simulink model "CF018A_GmRoadWhlInQlfr"  (R2013b)
settings: Solver=FixedStepDiscrete  SolverMode=SingleTasking  StartTime=0.0  StopTime=1  FixedStep=0.002  RelTol=1e-3
values from neighbouring files (symbols this model uses):
  DELTAPLSROLLOVR_CNT_S16 = DataDict.Constant    [CF018A_GmRoadWhlInQlfr_DataDict.m]
  DELTATISTAMPCNTROLLOVR_CNT_S32 = DataDict.Constant    [CF018A_GmRoadWhlInQlfr_DataDict.m]
  GmRoadWhlInQlfrMaxAllwblFrq = DataDict.Calibration    [CF018A_GmRoadWhlInQlfr_DataDict.m]
  GmRoadWhlInQlfrMaxFrqChg = DataDict.Calibration    [CF018A_GmRoadWhlInQlfr_DataDict.m]
  LEFRQCHGOUTOFRNG_CNT_U08 = DataDict.Constant    [CF018A_GmRoadWhlInQlfr_DataDict.m]
  LEFRQOUTOFRNG_CNT_U08 = DataDict.Constant    [CF018A_GmRoadWhlInQlfr_DataDict.m]
  NODEBSTEP_CNT_U16 = DataDict.Constant    [CF018A_GmRoadWhlInQlfr_DataDict.m]
  PARKDURN_CNT_F32 = DataDict.Constant    [CF018A_GmRoadWhlInQlfr_DataDict.m]
  PREVRAWWHLFRQMIN_HZ_F32 = DataDict.Constant    [CF018A_GmRoadWhlInQlfr_DataDict.m]
  RIFRQCHGOUTOFRNG_CNT_U08 = DataDict.Constant    [CF018A_GmRoadWhlInQlfr_DataDict.m]
  RIFRQOUTOFRNG_CNT_U08 = DataDict.Constant    [CF018A_GmRoadWhlInQlfr_DataDict.m]
  RoadWhlFrqInCalcOutOfRng = DataDict.NTC    [CF018A_GmRoadWhlInQlfr_DataDict.m]
  SECTO100MICROSECCNVN_CNT_F32 = DataDict.Constant    [CF018A_GmRoadWhlInQlfr_DataDict.m]
  WHLFRQMIN_HZ_F32 = DataDict.Constant    [CF018A_GmRoadWhlInQlfr_DataDict.m]
undefined symbols (not defined in the file or in its folder): NtcSts1
libraries: simulink x5, NxtrAbslt x2, NxtrLim x2
(part 1 of 5)
settings Model: PauseTimes=2  CovMetricSettings=dcmrw  CovFilter=CF09_GMOverlayStateHandler_v002_covfilter  CovHTMLOptions=-sRT=1 -aTS=1 -bRG=1 -bTC=1 -hTR=0 -nFC=0 -scm=1 -bcm=1 -xEv=0  covSaveCumulativeToWorkspaceVar=off  CovSaveSingleToWorkspaceVar=off  CovCumulativeReport=on  Creator=SZ7VY6  LastModifiedBy=BZHF94
settings SolverCC: AutoInsertRateTranBlk=on  InsertRTBMode=Always
settings DataIOCC: LimitDataPoints=off  SaveFormat=Structure  ReturnWorkspaceOutputs=on
settings OptimizationCC: BlockReduction=off  InlineParams=on  ZeroExternalMemoryAtStartup=off  ZeroInternalMemoryAtStartup=off  OptimizeModelRefInitCode=on  LifeSpan=1
settings DebuggingCC: SignalInfNanChecking=error  SignalRangeChecking=warning  UnderspecifiedInitializationDetection=Simplified  SolverPrmCheckMsg=error  InheritedTsInSrcMsg=error  DiscreteInheritContinuousMsg=error  SingleTaskRateTransMsg=error  TasksWithSamePriorityMsg=error  SigSpecEnsureSampleTimeMsg=error  CheckMatrixSingularityMsg=error  ParameterUnderflowMsg=error  ParameterPrecisionLossMsg=error  ParameterTunabilityLossMsg=error  FixptConstUnderflowMsg=warning  FixptConstOverflowMsg=warning  VectorMatrixConversionMsg=error  SignalLabelMismatchMsg=error  UnconnectedInputMsg=error  UnconnectedOutputMsg=error  UnconnectedLineMsg=error  SFcnCompatibilityMsg=error  UniqueDataStoreMsg=warning  BusObjectLabelMismatch=error  RootOutportRequireBusObject=error  AssertControl=DisableAll  ModelReferenceIOMsg=error  ModelReferenceVersionMismatchMessage=warning  ModelReferenceIOMismatchMessage=error  ModelReferenceCSMismatchMessage=warning  ModelReferenceDataLoggingMessage=error  StateNameClashWarn=warning  StrictBusMsg=ErrorOnBusTreatedAsVector  NonBusSignalsTreatedAsBus=error  SFUnexpectedBacktrackingDiag=error  SFInvalidInputDataAccessInChartInitDiag=error  SFNoUnconditionalDefaultTransitionDiag=error  SFTransitionOutsideNaturalParentDiag=error  SFUnconditionalTransitionShadowingDiag=error  SFUndirectedBroadcastEventsDiag=error
settings ModelReferenceCC: ModelReferenceNumInstancesAllowed=Single
settings RTWCC: SystemTargetFile=autosar.tlc  GenCodeOnly=on  TemplateMakefile=ert_default_tmf  Description=AUTOSAR  GenerateReport=on  ProcessScript=autosar_make_rtw_hook  LaunchReport=on
settings CodeAppCC: GenerateComments=off  IgnoreCustomStorageClasses=off  CustomSymbolStrType=$N$R$M  CustomSymbolStrBlkIO=$N$M  SimulinkBlockComments=off
settings STFCustomTargetCC: ParMdlRefBuildCompliant=on  CompOptLevelCompliant=on  IncludeMdlTerminateFcn=off  CombineOutputUpdateFcns=on  SuppressErrorStatus=on  ERTFirstTimeCompliant=on  ERTCustomFileBanners=on  SupportNonFinite=off  SupportComplex=off  SupportContinuousTime=off  SupportNonInlinedSFcns=off  MATLABClassNameForMDSCustomization=Simulink.SoftwareTarget.ERTCustomization  AutosarCompliant=on  GRTInterface=off  SystemTargetFile=autosar.tlc
settings ERTTargetCC: CodeReplacementLibrary=ANSI_C  ConcurrentExecutionCompliant=off  IncludeMdlTerminateFcn=off  SuppressErrorStatus=on  SupportNonFinite=off  SupportComplex=off  ModelStepFunctionPrototypeControlCompliant=off  CPPClassGenCompliant=off  AutosarCompliant=on  InlinedParameterPlacement=NonHierarchical  ERTCustomFileTemplate=example_file_process.tlc  EnableUserReplacementTypes=on

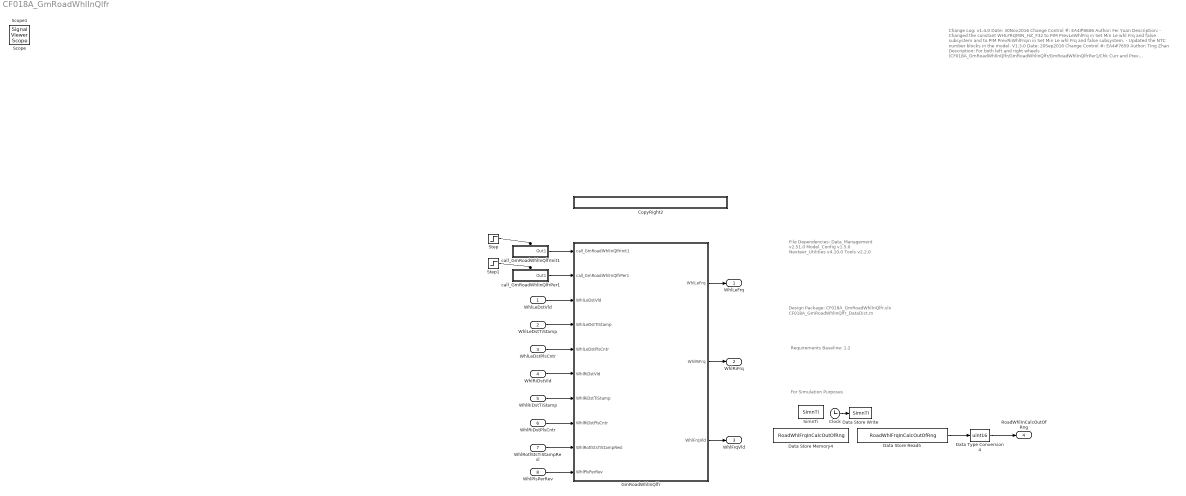
== system CF018A_GmRoadWhlInQlfr ==
  note: File Dependencies:
      |
      | Data_Management v2.51.0
      | Model_Config v1.5.0
      | Nexteer_Utilities v4.10.0
      | Tools v2.2.0
  note: Requirements Baseline: 1.2
  note: Change Log:
      |
      | v1.4.0
      | Date: 30Nov2016
      | Change Control #: EA4#8606
      | Author: Fei Yuan
      | Description:
      | - Changed the constant WHLFRQMIN_HZ_F32 to PIM PrevLeWhlFrq in
      |   Set Min Le whl Frq and false subsystem and to PIM PrevRiWhlFrqin  in
      |   Set Min Le whl Frq and false subsystem.
      | - Updated the NTC number blocks in the model.
      |
      |
      | V1.3.0
      | Date: 20Sep2016
      | Change Control #: EA4#7659
      | Author: Ting Zhan
      | Description:
      | For both left and right wheels (CF018A_GmRoadWhlInQlfr/GmRoadWhlInQlfr/GmRoadWhlInQlfrPer1/Chk Curr and Prev LeWhlDstTiStamp/Calc LeWhlFrq and LeWhlFrqVld /Calc
      | LeWhlFrq and LeWhlFrqVld and the corresponding right wheel block.)
      | 1.Adjust the math in the local processing functions to
      | cast to a sint32/sin16 before subtracting the timestampts/counters to produce the deltatistamp/deltacntr
      | 2.Move conversions before caluculating RawLeWhlFrq_WhlRevPerSec_T_F32 to avoid rollover
      |
      | V1.2.0
      | Date: 20Sep2016
      | Change Control #: EA4#4919
      | Author: Ting Zhan
      | Description:
      | -Added display variables dGmRoadWhlInQlrRawLeWhlFrq, dGmRoadWhlInQlrRawRiWhlFrq,
      |  dGmRoadWhlInQlrRawLeDeltaPls, dGmRoadWhlInQlrRawRiDeltaPls,
      |  dGmRoadWhlInQlrLeDeltaTiStamp, and dGmRoadWhlInQlrRiDeltaTiStamp
      | -Moved uint16 conversion after summation
      | -Changed time steps in .m file
      |
      | V 1.1.0
      | Date: 03Mar2016
      | Change Control #: EA4#7312
      | Author: Ting Zhan
      | Description:
      | - Added constant PREVRAWWHLFRQMIN_HZ_F32 in .m file
      |
      | V 1.0.0
      | Date: 22Feb2016
      | Change Control #: EA4#3951
      | Author: Ting Zhan
      | Description:
      | - Initial Release Based on EA4
      | CR Number: 3951
  note: For Simulation Purposes
  note: Design Package:
      | CF018A_GmRoadWhlInQlfr.slx
      | CF018A_GmRoadWhlInQlfr_DataDict.m
  WhlLeDstVld : Inport  RequirementInfo={} %GIDa_1b9c6812_2c02_4b85_9a2c_669458cc48bb  OutDataTypeStr=boolean
  WhlLeDstTiStamp : Inport  RequirementInfo={} %GIDa_61858a6e_79fe_432d_a90a_cf452097a93f  Port=2  OutDataTypeStr=uint16
  WhlLeDstPlsCntr : Inport  RequirementInfo={} %GIDa_f6a8d43a_8d7a_4621_b19c_bbf61fc3f1fb  Port=3  OutDataTypeStr=uint16
  WhlRiDstVld : Inport  RequirementInfo={} %GIDa_22f98033_b4f5_42bb_8f03_a53bfeb234c8  Port=4  OutDataTypeStr=boolean
  WhlRiDstTiStamp : Inport  RequirementInfo={} %GIDa_7d9397bd_97c2_42df_a94b_20b8f742e3e0  Port=5  OutDataTypeStr=uint16
  WhlRiDstPlsCntr : Inport  RequirementInfo={} %GIDa_8fb663a6_7a2b_45c8_868b_fc9c2da216fb  Port=6  OutDataTypeStr=uint16
  WhlRotlStsTiStampResl : Inport  RequirementInfo={} %GIDa_c41d293e_2c9d_4d75_aad1_09b36476f615  Port=7  OutDataTypeStr=single
  WhlPlsPerRev : Inport  RequirementInfo={} %GIDa_1e446983_1b59_4eb5_9ec1_824701f5829e  Port=8  OutDataTypeStr=uint8
  Clock : Clock
  CopyRight2 : Subsystem  Description=|  mask(Copyright Information){none=on}
      | Copyright info block.                                               
      |                                                                     
      | Place copyright information at the top of every subsystem in design.
      mask prompts: none "No parameters"
      mask help: Place copyright information at the top of every subsystem in design.
      mask Display:
      | NxtrConf = 'Nexteer Confidential';
      | 
      | sys = bdroot; %handle for the current model ("system")
      | first = get_param(sys,'Created');
      | if(isempty(first))
      |     first = datestr(now,'yyyy');
      | else
      |     first = first(end-3:end);  %year is last four digits
      | end
      | 
      | last = get_param(sys,'LastModifiedDate');
      | if isempty(last)
      |     last = datestr(now,'yyyy');
      | else
      |     last = last(end-3:end);
      | end
      | 
      | if strcmp(first,last)
      |     fprintf('%s -- Copyright %s Nexteer',NxtrConf,first)
      | else
      |     fprintf('%s -- %s%s- %s Nexteer',NxtrConf,char(169),first,last)
      | end
  Data Store Memory4 : DataStoreMemory  DataStoreName=RoadWhlFrqInCalcOutOfRng  InitialValue=NtcSts1.NTCSTS_PASSD  OutDataTypeStr=Enum: NtcSts1
  Data Store Read5 : DataStoreRead  DataStoreName=RoadWhlFrqInCalcOutOfRng  SampleTime=.004
  Data Store Write : DataStoreWrite  DataStoreName=SimnTi
  Data Type Conversion4 : DataTypeConversion  OutDataTypeStr=uint16
  GmRoadWhlInQlfr : Subsystem
  SimnTi : DataStoreMemory  DataStoreName=SimnTi
  Step : Step  Time=.001  Before=1  After=0  SampleTime=0
  Step1 : Step  Time=0.002  SampleTime=0
  call_GmRoadWhlInQlfrInit1 : Subsystem  TreatAsAtomicUnit=on
  call_GmRoadWhlInQlfrPer1 : Subsystem  TreatAsAtomicUnit=on
  WhlLeFrq : Outport  RequirementInfo={} %GIDa_1da87020_2114_47f8_bd6a_dcf122c70ef9
  WhlRiFrq : Outport  RequirementInfo={} %GIDa_aa71e542_5f04_4ff7_aa01_7ea85d72a732  Port=2
  WhlFrqVld : Outport  RequirementInfo={} %GIDa_6ce0db0a_f918_4040_a381_a66b37fb6372  Port=3
  RoadWhlInCalcOutOfRng : Outport  RequirementInfo={} %GIDa_f8f24313_b0b7_4842_bede_f0c570d36cae  Port=4
  Scope : SignalViewerScope  IOType=viewer  RefreshTime=0.035000
  Scope1 : SignalViewerScope  IOType=viewer  RefreshTime=0.035000
  wires:
  Step/1 -> call_GmRoadWhlInQlfrInit1/Enable
  call_GmRoadWhlInQlfrInit1/1(Out1) -> GmRoadWhlInQlfr/1(call_GmRoadWhlInQlfrInit1)
  Clock/1 -> Data Store Write/1
  GmRoadWhlInQlfr/2(WhlRiFrq) -> WhlRiFrq/1
  GmRoadWhlInQlfr/1(WhlLeFrq) -> WhlLeFrq/1
  Step1/1 -> call_GmRoadWhlInQlfrPer1/Enable
  call_GmRoadWhlInQlfrPer1/1(Out1) -> GmRoadWhlInQlfr/2(call_GmRoadWhlInQlfrPer1)
  GmRoadWhlInQlfr/3(WhlFrqVld) -> WhlFrqVld/1
  Data Store Read5/1 -> Data Type Conversion4/1
  Data Type Conversion4/1 -> RoadWhlInCalcOutOfRng/1
  WhlLeDstVld/1 -> GmRoadWhlInQlfr/3(WhlLeDstVld)
  WhlLeDstPlsCntr/1 -> GmRoadWhlInQlfr/5(WhlLeDstPlsCntr)
  WhlLeDstTiStamp/1 -> GmRoadWhlInQlfr/4(WhlLeDstTiStamp)
  WhlPlsPerRev/1 -> GmRoadWhlInQlfr/10(WhlPlsPerRev)
  WhlRiDstVld/1 -> GmRoadWhlInQlfr/6(WhlRiDstVld)
  WhlRiDstTiStamp/1 -> GmRoadWhlInQlfr/7(WhlRiDstTiStamp)
  WhlRiDstPlsCntr/1 -> GmRoadWhlInQlfr/8(WhlRiDstPlsCntr)
  WhlRotlStsTiStampResl/1 -> GmRoadWhlInQlfr/9(WhlRotlStsTiStampResl)

== system CF018A_GmRoadWhlInQlfr/CopyRight2 ==

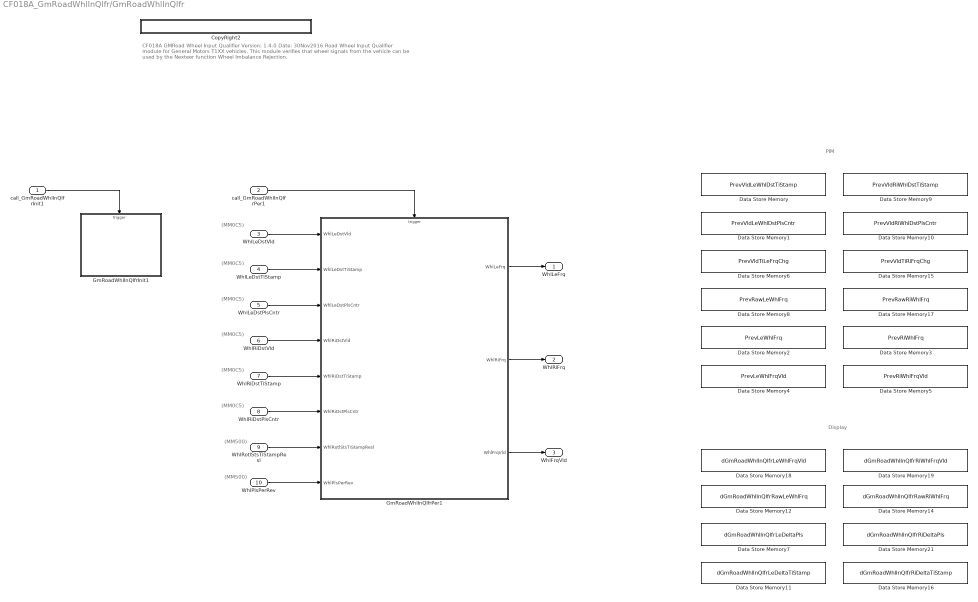
== system CF018A_GmRoadWhlInQlfr/GmRoadWhlInQlfr ==
  note: (MM0C5)
  note: CF018A  GMRoad Wheel Input Qualifier
      | Version: 1.4.0      Date: 30Nov2016
      |
      | Road Wheel Input Qualifier module for General Motors T1XX vehicles.
      | This module verifies that wheel signals from the vehicle can be used by the Nexteer function Wheel Imbalance Rejection.
  note: (MM500)
  note: (MM500)
  note: (MM0C5)
  note: (MM0C5)
  note: (MM0C5)
  note: (MM0C5)
  note: (MM0C5)
  note: PIM
  note: Display
  call_GmRoadWhlInQlfrInit1 : Inport  RequirementInfo={} %GIDa_bfdeb5c8_34d3_4847_8322_14533b8a1ec7
  call_GmRoadWhlInQlfrPer1 : Inport  RequirementInfo={} %GIDa_f1c70cb1_f5af_488b_94e7_678758a8a022  Port=2
  WhlLeDstVld : Inport  RequirementInfo="{'linktype_rmi_doors' '0000c6e7 (/GM T1XX/SubSystem Specifications/Customer Functions/CF018A GM Road Wheel Input Qualifier)' '#124' 'true' 'REQ:  124' '' } %GIDa_e1aceb09_ab93_45e7_ba05_ec3539382f7d"  Port=3
  WhlLeDstTiStamp : Inport  RequirementInfo="{'linktype_rmi_doors' '0000c6e7 (/GM T1XX/SubSystem Specifications/Customer Functions/CF018A GM Road Wheel Input Qualifier)' '#127' 'true' 'REQ:  127' '' } %GIDa_5b6463ec_722c_4fc4_9625_cb7f6c6361e1"  Port=4
  WhlLeDstPlsCntr : Inport  RequirementInfo="{'linktype_rmi_doors' '0000c6e7 (/GM T1XX/SubSystem Specifications/Customer Functions/CF018A GM Road Wheel Input Qualifier)' '#127' 'true' 'REQ:  127' '' } %GIDa_065f4aaa_928a_430a_bc48_84360d19c33c"  Port=5
  WhlRiDstVld : Inport  RequirementInfo="{'linktype_rmi_doors' '0000c6e7 (/GM T1XX/SubSystem Specifications/Customer Functions/CF018A GM Road Wheel Input Qualifier)' '#129' 'true' 'REQ:  129' '' } %GIDa_8d65498b_27df_4bf9_b0ab_bf83c8f9f21d"  Port=6
  WhlRiDstTiStamp : Inport  RequirementInfo="{'linktype_rmi_doors' '0000c6e7 (/GM T1XX/SubSystem Specifications/Customer Functions/CF018A GM Road Wheel Input Qualifier)' '#133' 'true' 'REQ:  133' '' } %GIDa_8ab7454d_6aff_452e_b449_8d99f946983c"  Port=7
  WhlRiDstPlsCntr : Inport  RequirementInfo="{'linktype_rmi_doors' '0000c6e7 (/GM T1XX/SubSystem Specifications/Customer Functions/CF018A GM Road Wheel Input Qualifier)' '#132' 'true' 'REQ:  132' '' } %GIDa_c4395fb0_b0ef_42d6_ba2f_71f5e37761ea"  Port=8
  WhlRotlStsTiStampResl : Inport  RequirementInfo="{'linktype_rmi_doors' '0000c6e7 (/GM T1XX/SubSystem Specifications/Customer Functions/CF018A GM Road Wheel Input Qualifier)' '#177' 'true' 'REQ:  177' '' } %GIDa_4023d9d2_72d9_498c_a3f9_a7c1df260df4"  Port=9
  WhlPlsPerRev : Inport  RequirementInfo="{'linktype_rmi_doors' '0000c6e7 (/GM T1XX/SubSystem Specifications/Customer Functions/CF018A GM Road Wheel Input Qualifier)' '#178' 'true' 'REQ:  178' '' } %GIDa_c7c8d484_f6c5_4f57_8e53_ca69660326b1"  Port=10
  CopyRight2 : Subsystem  Description=|  mask(Copyright Information){none=on}
      | Copyright info block.                                               
      |                                                                     
      | Place copyright information at the top of every subsystem in design.
      mask prompts: none "No parameters"
      mask help: Place copyright information at the top of every subsystem in design.
      mask Display:
      | NxtrConf = 'Nexteer Confidential';
      | 
      | sys = bdroot; %handle for the current model ("system")
      | first = get_param(sys,'Created');
      | if(isempty(first))
      |     first = datestr(now,'yyyy');
      | else
      |     first = first(end-3:end);  %year is last four digits
      | end
      | 
      | last = get_param(sys,'LastModifiedDate');
      | if isempty(last)
      |     last = datestr(now,'yyyy');
      | else
      |     last = last(end-3:end);
      | end
      | 
      | if strcmp(first,last)
      |     fprintf('%s -- Copyright %s Nexteer',NxtrConf,first)
      | else
      |     fprintf('%s -- %s%s- %s Nexteer',NxtrConf,char(169),first,last)
      | end
  Data Store Memory : DataStoreMemory  DataStoreName=PrevVldLeWhlDstTiStamp  InitialValue=[]  StateMustResolveToSignalObject=on
  Data Store Memory1 : DataStoreMemory  DataStoreName=PrevVldLeWhlDstPlsCntr  InitialValue=[]  StateMustResolveToSignalObject=on
  Data Store Memory10 : DataStoreMemory  DataStoreName=PrevVldRiWhlDstPlsCntr  InitialValue=[]  StateMustResolveToSignalObject=on
  Data Store Memory11 : DataStoreMemory  DataStoreName=dGmRoadWhlInQlfrLeDeltaTiStamp  InitialValue=[]  StateMustResolveToSignalObject=on
  Data Store Memory12 : DataStoreMemory  DataStoreName=dGmRoadWhlInQlfrRawLeWhlFrq  InitialValue=[]  StateMustResolveToSignalObject=on
  Data Store Memory14 : DataStoreMemory  DataStoreName=dGmRoadWhlInQlfrRawRiWhlFrq  InitialValue=[]  StateMustResolveToSignalObject=on
  Data Store Memory15 : DataStoreMemory  DataStoreName=PrevVldTiRiFrqChg  InitialValue=[]  StateMustResolveToSignalObject=on
  Data Store Memory16 : DataStoreMemory  DataStoreName=dGmRoadWhlInQlfrRiDeltaTiStamp  InitialValue=[]  StateMustResolveToSignalObject=on
  Data Store Memory17 : DataStoreMemory  DataStoreName=PrevRawRiWhlFrq  InitialValue=[]  StateMustResolveToSignalObject=on
  Data Store Memory18 : DataStoreMemory  DataStoreName=dGmRoadWhlInQlfrLeWhlFrqVld  InitialValue=[]  StateMustResolveToSignalObject=on
  Data Store Memory19 : DataStoreMemory  DataStoreName=dGmRoadWhlInQlfrRiWhlFrqVld  InitialValue=[]  StateMustResolveToSignalObject=on
  Data Store Memory2 : DataStoreMemory  DataStoreName=PrevLeWhlFrq  InitialValue=[]  StateMustResolveToSignalObject=on
  Data Store Memory21 : DataStoreMemory  DataStoreName=dGmRoadWhlInQlfrRiDeltaPls  InitialValue=[]  StateMustResolveToSignalObject=on
  Data Store Memory3 : DataStoreMemory  DataStoreName=PrevRiWhlFrq  InitialValue=[]  StateMustResolveToSignalObject=on
  Data Store Memory4 : DataStoreMemory  DataStoreName=PrevLeWhlFrqVld  InitialValue=[]  StateMustResolveToSignalObject=on
  Data Store Memory5 : DataStoreMemory  DataStoreName=PrevRiWhlFrqVld  InitialValue=[]  StateMustResolveToSignalObject=on
  Data Store Memory6 : DataStoreMemory  DataStoreName=PrevVldTiLeFrqChg  InitialValue=[]  StateMustResolveToSignalObject=on
  Data Store Memory7 : DataStoreMemory  DataStoreName=dGmRoadWhlInQlfrLeDeltaPls  InitialValue=[]  StateMustResolveToSignalObject=on
  Data Store Memory8 : DataStoreMemory  DataStoreName=PrevRawLeWhlFrq  InitialValue=[]  StateMustResolveToSignalObject=on
  Data Store Memory9 : DataStoreMemory  DataStoreName=PrevVldRiWhlDstTiStamp  InitialValue=[]  StateMustResolveToSignalObject=on
  GmRoadWhlInQlfrInit1 : Subsystem
  GmRoadWhlInQlfrPer1 : Subsystem
  WhlLeFrq : Outport  RequirementInfo="{'linktype_rmi_doors' '0000c6e7 (/GM T1XX/SubSystem Specifications/Customer Functions/CF018A GM Road Wheel Input Qualifier)' '#180' 'true' 'REQ:  180' '' } %GIDa_193ab0a0_dd30_4f7a_a182_b40d65e68801"
  WhlRiFrq : Outport  RequirementInfo="{'linktype_rmi_doors' '0000c6e7 (/GM T1XX/SubSystem Specifications/Customer Functions/CF018A GM Road Wheel Input Qualifier)' '#182' 'true' 'REQ:  182' '' } %GIDa_f59e91f0_fe76_4f29_916e_753e2c200ee2"  Port=2
  WhlFrqVld : Outport  RequirementInfo="{'linktype_rmi_doors' '0000c6e7 (/GM T1XX/SubSystem Specifications/Customer Functions/CF018A GM Road Wheel Input Qualifier)' '#181' 'true' 'REQ:  181' '' } %GIDa_2ee994e2_76da_417c_9ecc_5cdaff7fdb07"  Port=3
  wires:
  GmRoadWhlInQlfrPer1/2(WhlRiFrq) -> WhlRiFrq/1
  call_GmRoadWhlInQlfrPer1/1 -> GmRoadWhlInQlfrPer1/Trigger
  call_GmRoadWhlInQlfrInit1/1 -> GmRoadWhlInQlfrInit1/Trigger
  GmRoadWhlInQlfrPer1/1(WhlLeFrq) -> WhlLeFrq/1
  GmRoadWhlInQlfrPer1/3(WhlFrqVld) -> WhlFrqVld/1
  WhlLeDstVld/1 -> GmRoadWhlInQlfrPer1/1(WhlLeDstVld)
  WhlRiDstVld/1 -> GmRoadWhlInQlfrPer1/4(WhlRiDstVld)
  WhlRiDstPlsCntr/1 -> GmRoadWhlInQlfrPer1/6(WhlRiDstPlsCntr)
  WhlRiDstTiStamp/1 -> GmRoadWhlInQlfrPer1/5(WhlRiDstTiStamp)
  WhlRotlStsTiStampResl/1 -> GmRoadWhlInQlfrPer1/7(WhlRotlStsTiStampResl)
  WhlPlsPerRev/1 -> GmRoadWhlInQlfrPer1/8(WhlPlsPerRev)
  WhlLeDstPlsCntr/1 -> GmRoadWhlInQlfrPer1/3(WhlLeDstPlsCntr)
  WhlLeDstTiStamp/1 -> GmRoadWhlInQlfrPer1/2(WhlLeDstTiStamp)

== system CF018A_GmRoadWhlInQlfr/call_GmRoadWhlInQlfrInit1 ==
  Enable : EnablePort
  CopyRight2 : Subsystem  Description=|  mask(Copyright Information){none=on}
      | Copyright info block.                                               
      |                                                                     
      | Place copyright information at the top of every subsystem in design.
      mask prompts: none "No parameters"
      mask help: Place copyright information at the top of every subsystem in design.
      mask Display:
      | NxtrConf = 'Nexteer Confidential';
      | 
      | sys = bdroot; %handle for the current model ("system")
      | first = get_param(sys,'Created');
      | if(isempty(first))
      |     first = datestr(now,'yyyy');
      | else
      |     first = first(end-3:end);  %year is last four digits
      | end
      | 
      | last = get_param(sys,'LastModifiedDate');
      | if isempty(last)
      |     last = datestr(now,'yyyy');
      | else
      |     last = last(end-3:end);
      | end
      | 
      | if strcmp(first,last)
      |     fprintf('%s -- Copyright %s Nexteer',NxtrConf,first)
      | else
      |     fprintf('%s -- %s%s- %s Nexteer',NxtrConf,char(169),first,last)
      | end
  Function-Call Generator : simulink/Ports & Subsystems/Function-Call Generator  sample_time=.002  numberOfIterations=1
  Out1 : Outport
  wires:
  Function-Call Generator/1 -> Out1/1

== system CF018A_GmRoadWhlInQlfr/call_GmRoadWhlInQlfrPer1 ==
  Enable : EnablePort
  CopyRight2 : Subsystem  Description=|  mask(Copyright Information){none=on}
      | Copyright info block.                                               
      |                                                                     
      | Place copyright information at the top of every subsystem in design.
      mask prompts: none "No parameters"
      mask help: Place copyright information at the top of every subsystem in design.
      mask Display:
      | NxtrConf = 'Nexteer Confidential';
      | 
      | sys = bdroot; %handle for the current model ("system")
      | first = get_param(sys,'Created');
      | if(isempty(first))
      |     first = datestr(now,'yyyy');
      | else
      |     first = first(end-3:end);  %year is last four digits
      | end
      | 
      | last = get_param(sys,'LastModifiedDate');
      | if isempty(last)
      |     last = datestr(now,'yyyy');
      | else
      |     last = last(end-3:end);
      | end
      | 
      | if strcmp(first,last)
      |     fprintf('%s -- Copyright %s Nexteer',NxtrConf,first)
      | else
      |     fprintf('%s -- %s%s- %s Nexteer',NxtrConf,char(169),first,last)
      | end
  Function-Call Generator : simulink/Ports & Subsystems/Function-Call Generator  sample_time=.002  numberOfIterations=1
  Out1 : Outport
  wires:
  Function-Call Generator/1 -> Out1/1

== system CF018A_GmRoadWhlInQlfr/GmRoadWhlInQlfr/CopyRight2 ==

== system CF018A_GmRoadWhlInQlfr/GmRoadWhlInQlfr/GmRoadWhlInQlfrInit1 ==
  function : TriggerPort  TriggerType=function-call
  Constant1 : Constant  Value=WHLFRQMIN_HZ_F32  OutDataTypeStr=single
  Constant2 : Constant  Value=PREVRAWWHLFRQMIN_HZ_F32  OutDataTypeStr=single
  Constant3 : Constant  Value=WHLFRQMIN_HZ_F32  OutDataTypeStr=single
  Constant4 : Constant  Value=PREVRAWWHLFRQMIN_HZ_F32  OutDataTypeStr=single
  Constant5 : Constant  Value=RoadWhlFrqInCalcOutOfRng
  Constant7 : Constant  Value=NODEBSTEP_CNT_U16
  Constant8 : Constant  Value=0
  CopyRight2 : Subsystem  Description=|  mask(Copyright Information){none=on}
      | Copyright info block.                                               
      |                                                                     
      | Place copyright information at the top of every subsystem in design.
      mask prompts: none "No parameters"
      mask help: Place copyright information at the top of every subsystem in design.
      mask Display:
      | NxtrConf = 'Nexteer Confidential';
      | 
      | sys = bdroot; %handle for the current model ("system")
      | first = get_param(sys,'Created');
      | if(isempty(first))
      |     first = datestr(now,'yyyy');
      | else
      |     first = first(end-3:end);  %year is last four digits
      | end
      | 
      | last = get_param(sys,'LastModifiedDate');
      | if isempty(last)
      |     last = datestr(now,'yyyy');
      | else
      |     last = last(end-3:end);
      | end
      | 
      | if strcmp(first,last)
      |     fprintf('%s -- Copyright %s Nexteer',NxtrConf,first)
      | else
      |     fprintf('%s -- %s%s- %s Nexteer',NxtrConf,char(169),first,last)
      | end
  Data Store Write1 : DataStoreWrite  DataStoreName=PrevRiWhlFrq
      settings: AttributesFormatString=%<Priority>
  Data Store Write2 : DataStoreWrite  DataStoreName=PrevLeWhlFrq
      settings: AttributesFormatString=%<Priority>
  Data Store Write3 : DataStoreWrite  DataStoreName=PrevRawRiWhlFrq
      settings: AttributesFormatString=%<Priority>
  Data Store Write5 : DataStoreWrite  DataStoreName=PrevRawLeWhlFrq
      settings: AttributesFormatString=%<Priority>
  Enumerated Constant3 : simulink/Sources/Enumerated Constant  OutDataTypeStr=Enum: NtcSts1  Value=NtcSts1.NTCSTS_PASSD  SampleTime=inf
  NTC 0x0E3 Passd : Subsystem  mask(SetNTC){}
      mask help: SetNTC library block
  wires:
  Constant5/1 -> NTC 0x0E3 Passd/1(NtcNr)
  Enumerated Constant3/1 -> NTC 0x0E3 Passd/3(NtcSts)
  Constant7/1 -> NTC 0x0E3 Passd/4(DebStep)
  Constant8/1 -> NTC 0x0E3 Passd/2(NtcStInfo)
  Constant1/1 -> Data Store Write2/1
  Constant3/1 -> Data Store Write1/1
  Constant2/1 -> Data Store Write5/1
  Constant4/1 -> Data Store Write3/1

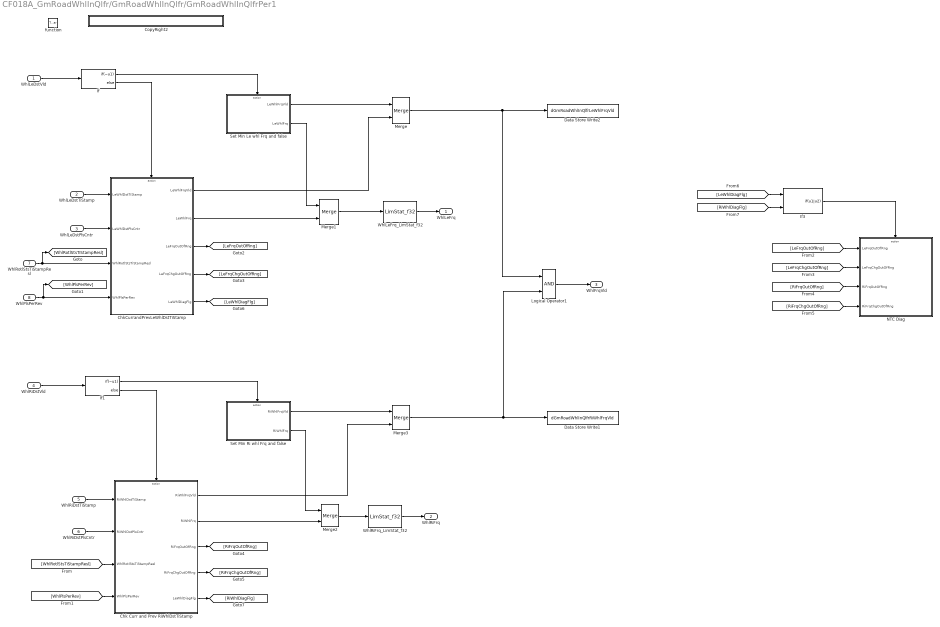
== system CF018A_GmRoadWhlInQlfr/GmRoadWhlInQlfr/GmRoadWhlInQlfrPer1 ==
  WhlLeDstVld : Inport  RequirementInfo="{'linktype_rmi_doors' '0000c6e7 (/GM T1XX/SubSystem Specifications/Customer Functions/CF018A GM Road Wheel Input Qualifier)' '#173' 'true' 'REQ:  173' '' ; 'linktype_rmi_doors' '0000c6e7 (/GM T1XX/SubSystem Specifications/Customer Functions/CF018A GM Road Wheel Input Qualifier)' '#174' 'true' 'REQ:  174' '' } %GIDa_d7700c8d_4dd2_4cfd_ada9_5810fd09f56e"
  WhlLeDstTiStamp : Inport  RequirementInfo="{'linktype_rmi_doors' '0000c6e7 (/GM T1XX/SubSystem Specifications/Customer Functions/CF018A GM Road Wheel Input Qualifier)' '#174' 'true' 'REQ:  174' '' } %GIDa_c64c8f74_dcbe_4ac4_8465_23f4747f243c"  Port=2
  WhlLeDstPlsCntr : Inport  RequirementInfo="{'linktype_rmi_doors' '0000c6e7 (/GM T1XX/SubSystem Specifications/Customer Functions/CF018A GM Road Wheel Input Qualifier)' '#174' 'true' 'REQ:  174' '' } %GIDa_615b43c0_e574_4964_9d11_9954a2d15f7a"  Port=3
  WhlRiDstVld : Inport  RequirementInfo="{'linktype_rmi_doors' '0000c6e7 (/GM T1XX/SubSystem Specifications/Customer Functions/CF018A GM Road Wheel Input Qualifier)' '#197' 'true' 'REQ:  197' '' ; 'linktype_rmi_doors' '0000c6e7 (/GM T1XX/SubSystem Specifications/Customer Functions/CF018A GM Road Wheel Input Qualifier)' '#184' 'true' 'REQ:  184' '' } %GIDa_4b773b89_db55_4f6d_8b97_064fbe3148f1"  Port=4
  WhlRiDstTiStamp : Inport  RequirementInfo="{'linktype_rmi_doors' '0000c6e7 (/GM T1XX/SubSystem Specifications/Customer Functions/CF018A GM Road Wheel Input Qualifier)' '#184' 'true' 'REQ:  184' '' } %GIDa_a3db22bf_c8b4_41b0_aa50_279e52724179"  Port=5
  WhlRiDstPlsCntr : Inport  RequirementInfo="{'linktype_rmi_doors' '0000c6e7 (/GM T1XX/SubSystem Specifications/Customer Functions/CF018A GM Road Wheel Input Qualifier)' '#184' 'true' 'REQ:  184' '' } %GIDa_b60c6f9e_af98_4dd6_8968_245fbd651cfc"  Port=6
  WhlRotlStsTiStampResl : Inport  RequirementInfo="{'linktype_rmi_doors' '0000c6e7 (/GM T1XX/SubSystem Specifications/Customer Functions/CF018A GM Road Wheel Input Qualifier)' '#174' 'true' 'REQ:  174' '' } %GIDa_91c21ce4_69c5_4031_9a49_c9101c1f4761"  Port=7
  WhlPlsPerRev : Inport  RequirementInfo="{'linktype_rmi_doors' '0000c6e7 (/GM T1XX/SubSystem Specifications/Customer Functions/CF018A GM Road Wheel Input Qualifier)' '#174' 'true' 'REQ:  174' '' } %GIDa_72373332_7f32_4578_a651_18486be9e00f"  Port=8
  function : TriggerPort  TriggerType=function-call
  Chk Curr and Prev RiWhlDstTiStamp : Subsystem  RequirementInfo="{'linktype_rmi_doors' '0000c6e7 (/GM T1XX/SubSystem Specifications/Customer Functions/CF018A GM Road Wheel Input Qualifier)' '#184' 'true' 'REQ:  184' '' } %GIDa_2041cd56_69f4_48ea_af70_933be3b3db5a"  TreatAsAtomicUnit=on
  ChkCurrandPrevLeWhlDstTiStamp : Subsystem  RequirementInfo="{'linktype_rmi_doors' '0000c6e7 (/GM T1XX/SubSystem Specifications/Customer Functions/CF018A GM Road Wheel Input Qualifier)' '#174' 'true' 'REQ:  174' '' } %GIDa_0b29a29f_8e1d_448a_a108_8e8795f569a4"  TreatAsAtomicUnit=on
  CopyRight2 : Subsystem  Description=|  mask(Copyright Information){none=on}
      | Copyright info block.                                               
      |                                                                     
      | Place copyright information at the top of every subsystem in design.
      mask prompts: none "No parameters"
      mask help: Place copyright information at the top of every subsystem in design.
      mask Display:
      | NxtrConf = 'Nexteer Confidential';
      | 
      | sys = bdroot; %handle for the current model ("system")
      | first = get_param(sys,'Created');
      | if(isempty(first))
      |     first = datestr(now,'yyyy');
      | else
      |     first = first(end-3:end);  %year is last four digits
      | end
      | 
      | last = get_param(sys,'LastModifiedDate');
      | if isempty(last)
      |     last = datestr(now,'yyyy');
      | else
      |     last = last(end-3:end);
      | end
      | 
      | if strcmp(first,last)
      |     fprintf('%s -- Copyright %s Nexteer',NxtrConf,first)
      | else
      |     fprintf('%s -- %s%s- %s Nexteer',NxtrConf,char(169),first,last)
      | end
  Data Store Write1 : DataStoreWrite  DataStoreName=dGmRoadWhlInQlfrRiWhlFrqVld
  Data Store Write2 : DataStoreWrite  DataStoreName=dGmRoadWhlInQlfrLeWhlFrqVld
  If : If  RequirementInfo="{'linktype_rmi_doors' '0000c6e7 (/GM T1XX/SubSystem Specifications/Customer Functions/CF018A GM Road Wheel Input Qualifier)' '#173' 'true' 'REQ:  173' '' ; 'linktype_rmi_doors' '0000c6e7 (/GM T1XX/SubSystem Specifications/Customer Functions/CF018A GM Road Wheel Input Qualifier)' '#174' 'true' 'REQ:  174' '' } %GIDa_d4101963_70fa_4f69_9d60_52bbea4bf737"  IfExpression=~u1
      settings: AttributesFormatString=%<Priority>
  If1 : If  RequirementInfo="{'linktype_rmi_doors' '0000c6e7 (/GM T1XX/SubSystem Specifications/Customer Functions/CF018A GM Road Wheel Input Qualifier)' '#197' 'true' 'REQ:  197' '' ; 'linktype_rmi_doors' '0000c6e7 (/GM T1XX/SubSystem Specifications/Customer Functions/CF018A GM Road Wheel Input Qualifier)' '#184' 'true' 'REQ:  184' '' } %GIDa_770ddd54_bfa9_4385_a59f_751f7eeeab56"  IfExpression=~u1
      settings: AttributesFormatString=%<Priority>
  If3 : If  RequirementInfo="{'linktype_rmi_doors' '0000c6e7 (/GM T1XX/SubSystem Specifications/Customer Functions/CF018A GM Road Wheel Input Qualifier)' '#53' 'true' 'REQ:  53' '' } %GIDa_fb051f22_4249_4689_b92e_ba64f9372af6"  NumInputs=2  IfExpression=u1|u2  ShowElse=off
  Logical Operator1 : Logic  AllPortsSameDT=off  OutDataTypeStr=boolean
  Merge : Merge  RequirementInfo="{'linktype_rmi_doors' '0000c6e7 (/GM T1XX/SubSystem Specifications/Customer Functions/CF018A GM Road Wheel Input Qualifier)' '#173' 'true' 'REQ:  173' '' } %GIDa_cb002f7a_b7be_4f45_aac1_af736668bf4c"
  Merge1 : Merge  RequirementInfo="{'linktype_rmi_doors' '0000c6e7 (/GM T1XX/SubSystem Specifications/Customer Functions/CF018A GM Road Wheel Input Qualifier)' '#174' 'true' 'REQ:  174' '' } %GIDa_ddccbc5e_b156_435f_975e_435c2cbc9a07"
  Merge2 : Merge  RequirementInfo="{'linktype_rmi_doors' '0000c6e7 (/GM T1XX/SubSystem Specifications/Customer Functions/CF018A GM Road Wheel Input Qualifier)' '#197' 'true' 'REQ:  197' '' ; 'linktype_rmi_doors' '0000c6e7 (/GM T1XX/SubSystem Specifications/Customer Functions/CF018A GM Road Wheel Input Qualifier)' '#184' 'true' 'REQ:  184' '' } %GIDa_9ea871d5_0a76_4537_8167_96f8acf61823"
  Merge3 : Merge  RequirementInfo="{'linktype_rmi_doors' '0000c6e7 (/GM T1XX/SubSystem Specifications/Customer Functions/CF018A GM Road Wheel Input Qualifier)' '#197' 'true' 'REQ:  197' '' ; 'linktype_rmi_doors' '0000c6e7 (/GM T1XX/SubSystem Specifications/Customer Functions/CF018A GM Road Wheel Input Qualifier)' '#184' 'true' 'REQ:  184' '' } %GIDa_9dc5d5e1_26ec_4822_b43e_9012cab3bf3b"
  NTC Diag : Subsystem  RequirementInfo="{'linktype_rmi_doors' '0000c6e7 (/GM T1XX/SubSystem Specifications/Customer Functions/CF018A GM Road Wheel Input Qualifier)' '#53' 'true' 'REQ:  53' '' } %GIDa_58a28ebd_950b_4c57_bce1_ae0243545563"  TreatAsAtomicUnit=on
  "Set Min Le whl Frq and false " : Subsystem  RequirementInfo="{'linktype_rmi_doors' '0000c6e7 (/GM T1XX/SubSystem Specifications/Customer Functions/CF018A GM Road Wheel Input Qualifier)' '#173' 'true' 'REQ:  173' '' } %GIDa_9a0c942b_82ca_49bc_8677_cad5c258b403"  TreatAsAtomicUnit=on
  "Set Min Ri whl Frq and false " : Subsystem  RequirementInfo="{'linktype_rmi_doors' '0000c6e7 (/GM T1XX/SubSystem Specifications/Customer Functions/CF018A GM Road Wheel Input Qualifier)' '#197' 'true' 'REQ:  197' '' } %GIDa_06425b0c_0cdb_41d8_84f9_853563edc118"  TreatAsAtomicUnit=on
  WhlLeFrq_LimStat_f32 : NxtrLim/LimStat_f32  RequirementInfo="{'linktype_rmi_doors' '0000c6e7 (/GM T1XX/SubSystem Specifications/Customer Functions/CF018A GM Road Wheel Input Qualifier)' '#174' 'true' 'REQ:  174' '' } %GIDa_6ee6fd7b_4fe2_4ec5_b756_c35f52ef8779"  LoLim=WHLFRQMIN_HZ_F32  HiLim=WHLFRQMAX_HZ_F32
      settings: AttributesFormatString=|
      | Low Limit: %<LoLim>
      | High Limit:%<HiLim>
  WhlRiFrq_LimStat_f32 : NxtrLim/LimStat_f32  RequirementInfo="{'linktype_rmi_doors' '0000c6e7 (/GM T1XX/SubSystem Specifications/Customer Functions/CF018A GM Road Wheel Input Qualifier)' '#197' 'true' 'REQ:  197' '' ; 'linktype_rmi_doors' '0000c6e7 (/GM T1XX/SubSystem Specifications/Customer Functions/CF018A GM Road Wheel Input Qualifier)' '#184' 'true' 'REQ:  184' '' } %GIDa_ef4aac55_22ec_438e_bc70_4b32bc6e8131"  LoLim=WHLFRQMIN_HZ_F32  HiLim=WHLFRQMAX_HZ_F32
      settings: AttributesFormatString=|
      | Low Limit: %<LoLim>
      | High Limit:%<HiLim>
  WhlLeFrq : Outport  RequirementInfo="{'linktype_rmi_doors' '0000c6e7 (/GM T1XX/SubSystem Specifications/Customer Functions/CF018A GM Road Wheel Input Qualifier)' '#174' 'true' 'REQ:  174' '' } %GIDa_ad72c3fe_3139_49da_a979_17fad9a56d26"
  WhlRiFrq : Outport  RequirementInfo="{'linktype_rmi_doors' '0000c6e7 (/GM T1XX/SubSystem Specifications/Customer Functions/CF018A GM Road Wheel Input Qualifier)' '#197' 'true' 'REQ:  197' '' ; 'linktype_rmi_doors' '0000c6e7 (/GM T1XX/SubSystem Specifications/Customer Functions/CF018A GM Road Wheel Input Qualifier)' '#184' 'true' 'REQ:  184' '' } %GIDa_d612d29e_15cf_4b34_a52b_3ad5f32a3424"  Port=2
  WhlFrqVld : Outport  RequirementInfo={} %GIDa_4f5ed7b0_e7c7_4643_be2f_11317918436d  Port=3
  wires:
  WhlRiFrq_LimStat_f32/1 -> WhlRiFrq/1
  WhlLeDstVld/1 -> If/1
  If/1 -> "Set Min Le whl Frq and false "/Action
  If/2 -> ChkCurrandPrevLeWhlDstTiStamp/Action
  WhlLeDstTiStamp/1 -> ChkCurrandPrevLeWhlDstTiStamp/1(LeWhlDstTiStamp)
  WhlLeDstPlsCntr/1 -> ChkCurrandPrevLeWhlDstTiStamp/2(LeWhlDstPlsCntr)
  WhlRotlStsTiStampResl/1 -> [WhlRotlStsTiStampResl], ChkCurrandPrevLeWhlDstTiStamp/3(WhlRotlStsTiStampResl)
  WhlPlsPerRev/1 -> [WhlPlsPerRev], ChkCurrandPrevLeWhlDstTiStamp/4(WhlPlsPerRev)
  ChkCurrandPrevLeWhlDstTiStamp/1(LeWhlFrqVld) -> Merge/2
  "Set Min Le whl Frq and false "/1(LeWhlFrqVld) -> Merge/1
  "Set Min Le whl Frq and false "/2(LeWhlFrq) -> Merge1/1
  ChkCurrandPrevLeWhlDstTiStamp/2(LeWhlFrq) -> Merge1/2
  WhlRiDstVld/1 -> If1/1
  WhlRiDstPlsCntr/1 -> Chk Curr and Prev RiWhlDstTiStamp/2(RiWhlDstPlsCntr)
  WhlRiDstTiStamp/1 -> Chk Curr and Prev RiWhlDstTiStamp/1(RiWhlDstTiStamp)
  If1/1 -> "Set Min Ri whl Frq and false "/Action
  If1/2 -> Chk Curr and Prev RiWhlDstTiStamp/Action
  Chk Curr and Prev RiWhlDstTiStamp/1(RiWhlFrqVld) -> Merge3/2
  "Set Min Ri whl Frq and false "/1(RiWhlFrqVld) -> Merge3/1
  [WhlRotlStsTiStampResl] -> Chk Curr and Prev RiWhlDstTiStamp/3(WhlRotlStsTiStampResl)
  [WhlPlsPerRev] -> Chk Curr and Prev RiWhlDstTiStamp/4(WhlPlsPerRev)
  "Set Min Ri whl Frq and false "/2(RiWhlFrq) -> Merge2/1
  Chk Curr and Prev RiWhlDstTiStamp/2(RiWhlFrq) -> Merge2/2
  Merge1/1 -> WhlLeFrq_LimStat_f32/1
  Merge2/1 -> WhlRiFrq_LimStat_f32/1
  Logical Operator1/1 -> WhlFrqVld/1
  Merge/1 -> Logical Operator1/1, Data Store Write2/1
  WhlLeFrq_LimStat_f32/1 -> WhlLeFrq/1
  ChkCurrandPrevLeWhlDstTiStamp/3(LeFrqOutOfRng) -> [LeFrqOutOfRng]
  ChkCurrandPrevLeWhlDstTiStamp/4(LeFrqChgOutOfRng) -> [LeFrqChgOutOfRng]
  Chk Curr and Prev RiWhlDstTiStamp/3(RiFrqOutOfRng) -> [RiFrqOutOfRng]
  Chk Curr and Prev RiWhlDstTiStamp/4(RiFrqChgOutOfRng) -> [RiFrqChgOutOfRng]
  If3/1 -> NTC Diag/Action
  ChkCurrandPrevLeWhlDstTiStamp/5(LeWhlDiagFlg) -> [LeWhlDiagFlg]
  [LeWhlDiagFlg] -> If3/1
  [RiWhlDiagFlg] -> If3/2
  Chk Curr and Prev RiWhlDstTiStamp/5(LeWhlDiagFlg) -> [RiWhlDiagFlg]
  [LeFrqOutOfRng] -> NTC Diag/1(LeFrqOutOfRng)
  [LeFrqChgOutOfRng] -> NTC Diag/2(LeFrqChgOutOfRng)
  [RiFrqOutOfRng] -> NTC Diag/3(RiFrqOutOfRng)
  [RiFrqChgOutOfRng] -> NTC Diag/4(RiFrqChgOutOfRng)
  Merge3/1 -> Data Store Write1/1, Logical Operator1/2

== system CF018A_GmRoadWhlInQlfr/call_GmRoadWhlInQlfrInit1/CopyRight2 ==

== system CF018A_GmRoadWhlInQlfr/call_GmRoadWhlInQlfrPer1/CopyRight2 ==

== system CF018A_GmRoadWhlInQlfr/GmRoadWhlInQlfr/GmRoadWhlInQlfrInit1/CopyRight2 ==

== system CF018A_GmRoadWhlInQlfr/GmRoadWhlInQlfr/GmRoadWhlInQlfrInit1/NTC 0x0E3 Passd ==
  NtcNr : Inport
  NtcStInfo : Inport  Port=2
  NtcSts : Inport  Port=3
  DebStep : Inport  Port=4
  SetNtcSts : Subsystem  RequirementInfo={} %GIDa_bb35cd0f_967e_4660_bcc8_350a5453475d  TreatAsAtomicUnit=on
      settings: RTWSystemCode=Inline
  wires:
  NtcStInfo/1 -> SetNtcSts/2(NtcStInfo)
  DebStep/1 -> SetNtcSts/4(DebStep)
  NtcSts/1 -> SetNtcSts/3(NtcSts)
  NtcNr/1 -> SetNtcSts/1(NtcNr)  "NtcNr"

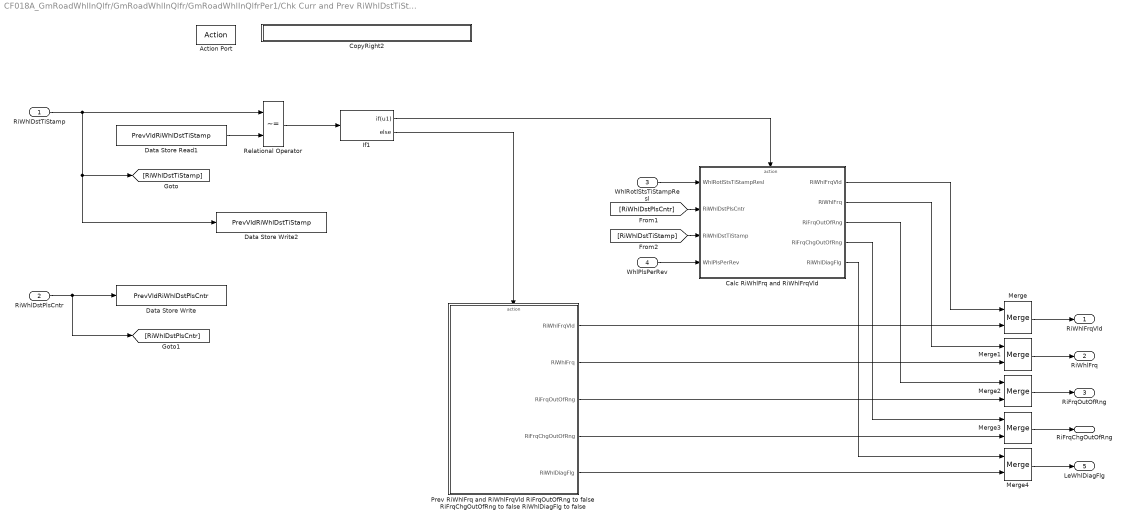
== system CF018A_GmRoadWhlInQlfr/GmRoadWhlInQlfr/GmRoadWhlInQlfrPer1/Chk Curr and Prev RiWhlDstTiStamp ==
  RiWhlDstTiStamp : Inport  RequirementInfo="{'linktype_rmi_doors' '0000c6e7 (/GM T1XX/SubSystem Specifications/Customer Functions/CF018A GM Road Wheel Input Qualifier)' '#184' 'true' 'REQ:  184' '' ; 'linktype_rmi_doors' '0000c6e7 (/GM T1XX/SubSystem Specifications/Customer Functions/CF018A GM Road Wheel Input Qualifier)' '#187' 'true' 'REQ:  187' '' } %GIDa_6d507ec8_8554_4974_b316_4b32989dfd14"
  RiWhlDstPlsCntr : Inport  RequirementInfo="{'linktype_rmi_doors' '0000c6e7 (/GM T1XX/SubSystem Specifications/Customer Functions/CF018A GM Road Wheel Input Qualifier)' '#184' 'true' 'REQ:  184' '' } %GIDa_b91254f7_d06e_406c_b1d8_e46fe3b22d44"  Port=2
  WhlRotlStsTiStampResl : Inport  RequirementInfo="{'linktype_rmi_doors' '0000c6e7 (/GM T1XX/SubSystem Specifications/Customer Functions/CF018A GM Road Wheel Input Qualifier)' '#187' 'true' 'REQ:  187' '' } %GIDa_91492a28_296c_44fe_99fd_f764f535019b"  Port=3
  WhlPlsPerRev : Inport  RequirementInfo="{'linktype_rmi_doors' '0000c6e7 (/GM T1XX/SubSystem Specifications/Customer Functions/CF018A GM Road Wheel Input Qualifier)' '#187' 'true' 'REQ:  187' '' } %GIDa_b73c1771_1231_4786_aa6a_a054164eaf89"  Port=4
  Action Port : ActionPort  ActionType=else
  "Calc RiWhlFrq and RiWhlFrqVld " : Subsystem  RequirementInfo="{'linktype_rmi_doors' '0000c6e7 (/GM T1XX/SubSystem Specifications/Customer Functions/CF018A GM Road Wheel Input Qualifier)' '#187' 'true' 'REQ:  187' '' } %GIDa_3af1f4fc_b3d2_4e47_a3fb_14e01ae22a95"  TreatAsAtomicUnit=on
      settings: AttributesFormatString=%<Priority>
  CopyRight2 : Subsystem  Description=|  mask(Copyright Information){none=on}
      | Copyright info block.                                               
      |                                                                     
      | Place copyright information at the top of every subsystem in design.
      mask prompts: none "No parameters"
      mask help: Place copyright information at the top of every subsystem in design.
      mask Display:
      | NxtrConf = 'Nexteer Confidential';
      | 
      | sys = bdroot; %handle for the current model ("system")
      | first = get_param(sys,'Created');
      | if(isempty(first))
      |     first = datestr(now,'yyyy');
      | else
      |     first = first(end-3:end);  %year is last four digits
      | end
      | 
      | last = get_param(sys,'LastModifiedDate');
      | if isempty(last)
      |     last = datestr(now,'yyyy');
      | else
      |     last = last(end-3:end);
      | end
      | 
      | if strcmp(first,last)
      |     fprintf('%s -- Copyright %s Nexteer',NxtrConf,first)
      | else
      |     fprintf('%s -- %s%s- %s Nexteer',NxtrConf,char(169),first,last)
      | end
  Data Store Read1 : DataStoreRead  RequirementInfo="{'linktype_rmi_doors' '0000c6e7 (/GM T1XX/SubSystem Specifications/Customer Functions/CF018A GM Road Wheel Input Qualifier)' '#184' 'true' 'REQ:  184' '' ; 'linktype_rmi_doors' '0000c6e7 (/GM T1XX/SubSystem Specifications/Customer Functions/CF018A GM Road Wheel Input Qualifier)' '#187' 'true' 'REQ:  187' '' } %GIDa_f94b6e77_1e08_44dc_ba8d_ad47bd5666eb"  Priority=0  DataStoreName=PrevVldRiWhlDstTiStamp
      settings: AttributesFormatString=%<Priority>
  Data Store Write : DataStoreWrite  RequirementInfo="{'linktype_rmi_doors' '0000c6e7 (/GM T1XX/SubSystem Specifications/Customer Functions/CF018A GM Road Wheel Input Qualifier)' '#184' 'true' 'REQ:  184' '' } %GIDa_57ebfaa4_d586_44a7_b211_025fb3bce2fc"  Priority=2  DataStoreName=PrevVldRiWhlDstPlsCntr
      settings: AttributesFormatString=%<Priority>
  Data Store Write2 : DataStoreWrite  RequirementInfo="{'linktype_rmi_doors' '0000c6e7 (/GM T1XX/SubSystem Specifications/Customer Functions/CF018A GM Road Wheel Input Qualifier)' '#184' 'true' 'REQ:  184' '' } %GIDa_fe8d1ae2_0082_4fe0_8a55_4cd734f4cf10"  Priority=2  DataStoreName=PrevVldRiWhlDstTiStamp
      settings: AttributesFormatString=%<Priority>
  If1 : If  RequirementInfo="{'linktype_rmi_doors' '0000c6e7 (/GM T1XX/SubSystem Specifications/Customer Functions/CF018A GM Road Wheel Input Qualifier)' '#187' 'true' 'REQ:  187' '' } %GIDa_e984f34a_6592_44c2_8b53_0c9e11f32243"  Priority=1  IfExpression=u1
      settings: AttributesFormatString=%<Priority>
  Merge{,1..4} (5 alike) : Merge
  "Prev RiWhlFrq and RiWhlFrqVld RiFrqOutOfRng to false RiFrqChgOutOfRng to false RiWhlDiagFlg to false " : Subsystem  RequirementInfo="{'linktype_rmi_doors' '0000c6e7 (/GM T1XX/SubSystem Specifications/Customer Functions/CF018A GM Road Wheel Input Qualifier)' '#184' 'true' 'REQ:  184' '' } %GIDa_0630611b_2d83_40f3_b140_82be7320c2e7"  TreatAsAtomicUnit=on
  Relational Operator : RelationalOperator  RequirementInfo="{'linktype_rmi_doors' '0000c6e7 (/GM T1XX/SubSystem Specifications/Customer Functions/CF018A GM Road Wheel Input Qualifier)' '#184' 'true' 'REQ:  184' '' ; 'linktype_rmi_doors' '0000c6e7 (/GM T1XX/SubSystem Specifications/Customer Functions/CF018A GM Road Wheel Input Qualifier)' '#187' 'true' 'REQ:  187' '' } %GIDa_500e532e_b250_4068_9932_efc74e0a085c"  Operator=~=  OutDataTypeStr=boolean
  RiWhlFrqVld : Outport
  RiWhlFrq : Outport  Port=2
  RiFrqOutOfRng : Outport  Port=3
  RiFrqChgOutOfRng : Outport  Port=4
  LeWhlDiagFlg : Outport  Port=5
  wires:
  WhlPlsPerRev/1 -> "Calc RiWhlFrq and RiWhlFrqVld "/4(WhlPlsPerRev)
  [RiWhlDstTiStamp] -> "Calc RiWhlFrq and RiWhlFrqVld "/3(RiWhlDstTiStamp)
  [RiWhlDstPlsCntr] -> "Calc RiWhlFrq and RiWhlFrqVld "/2(RiWhlDstPlsCntr)
  RiWhlDstPlsCntr/1 -> Data Store Write/1, [RiWhlDstPlsCntr]
  WhlRotlStsTiStampResl/1 -> "Calc RiWhlFrq and RiWhlFrqVld "/1(WhlRotlStsTiStampResl)
  RiWhlDstTiStamp/1 -> Relational Operator/1, [RiWhlDstTiStamp], Data Store Write2/1
  Data Store Read1/1 -> Relational Operator/2
  If1/1 -> "Calc RiWhlFrq and RiWhlFrqVld "/Action
  Relational Operator/1 -> If1/1
  "Prev RiWhlFrq and RiWhlFrqVld RiFrqOutOfRng to false RiFrqChgOutOfRng to false RiWhlDiagFlg to false "/4(RiFrqChgOutOfRng) -> Merge3/2
  "Prev RiWhlFrq and RiWhlFrqVld RiFrqOutOfRng to false RiFrqChgOutOfRng to false RiWhlDiagFlg to false "/3(RiFrqOutOfRng) -> Merge2/2
  "Prev RiWhlFrq and RiWhlFrqVld RiFrqOutOfRng to false RiFrqChgOutOfRng to false RiWhlDiagFlg to false "/2(RiWhlFrq) -> Merge1/2
  "Prev RiWhlFrq and RiWhlFrqVld RiFrqOutOfRng to false RiFrqChgOutOfRng to false RiWhlDiagFlg to false "/1(RiWhlFrqVld) -> Merge/2
  Merge/1 -> RiWhlFrqVld/1
  Merge1/1 -> RiWhlFrq/1
  Merge2/1 -> RiFrqOutOfRng/1
  Merge3/1 -> RiFrqChgOutOfRng/1
  If1/2 -> "Prev RiWhlFrq and RiWhlFrqVld RiFrqOutOfRng to false RiFrqChgOutOfRng to false RiWhlDiagFlg to false "/Action
  "Calc RiWhlFrq and RiWhlFrqVld "/2(RiWhlFrq) -> Merge1/1
  "Calc RiWhlFrq and RiWhlFrqVld "/1(RiWhlFrqVld) -> Merge/1
  "Calc RiWhlFrq and RiWhlFrqVld "/3(RiFrqOutOfRng) -> Merge2/1
  "Calc RiWhlFrq and RiWhlFrqVld "/4(RiFrqChgOutOfRng) -> Merge3/1
  "Prev RiWhlFrq and RiWhlFrqVld RiFrqOutOfRng to false RiFrqChgOutOfRng to false RiWhlDiagFlg to false "/5(RiWhlDiagFlg) -> Merge4/2
  Merge4/1 -> LeWhlDiagFlg/1
  "Calc RiWhlFrq and RiWhlFrqVld "/5(RiWhlDiagFlg) -> Merge4/1
